simulink model "Zadanie5"  (Simulink 7.5)
settings: Solver=ode4  StartTime=0.0  StopTime=10.0  FixedStep=0.01  RelTol=1e-3
settings Model: Creator=coder89  LastModifiedBy=coder89

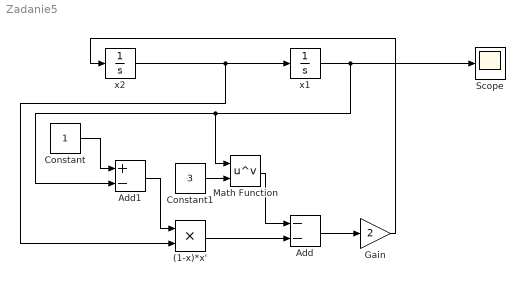
== system Zadanie5 ==
  (1-x)*x' : Product  OutDataType=fixdt(1, 16)  OutScaling=2^0  RndMeth=Zero
  Add : Sum  Inputs=--  OutDataType=fixdt(1, 16)  OutScaling=2^-10
  Add1 : Sum  Inputs=+-  OutDataType=fixdt(1, 16)  OutScaling=2^-10
  Constant : Constant  OutDataType=fixdt(1, 16)  OutScaling=2^0
  Constant1 : Constant  Value=3  OutDataType=fixdt(1, 16)  OutScaling=2^0
  Gain : Gain  Gain=2  ParameterDataType=fixdt(1, 16)  ParameterScaling=2^0  OutDataType=fixdt(1, 16)  OutScaling=2^0
  Math Function : Math  Operator=pow  OutputSignalType=real  OutDataType=fixdt(1, 16)  OutScaling=2^0  SaturateOnIntegerOverflow=on
  Scope : Scope
  x1 : Integrator  InitialCondition=21
  x2 : Integrator  InitialCondition=30
  wires:
  x2/1 -> x1/1, (1-x)*x'/2
  x1/1 -> Add1/2, Math Function/1, Scope/1
  Constant/1 -> Add1/1
  Math Function/1 -> Add/1
  (1-x)*x'/1 -> Add/2
  Add1/1 -> (1-x)*x'/1
  Add/1 -> Gain/1
  Gain/1 -> x2/1
  Constant1/1 -> Math Function/2
